simulink model "pillow"  (Simulink 7.0)
settings: Solver=ode45  StartTime=0.0  StopTime=10.0  RelTol=1e-3
settings Model: Creator=FHUANG  LastModifiedBy=FHUANG

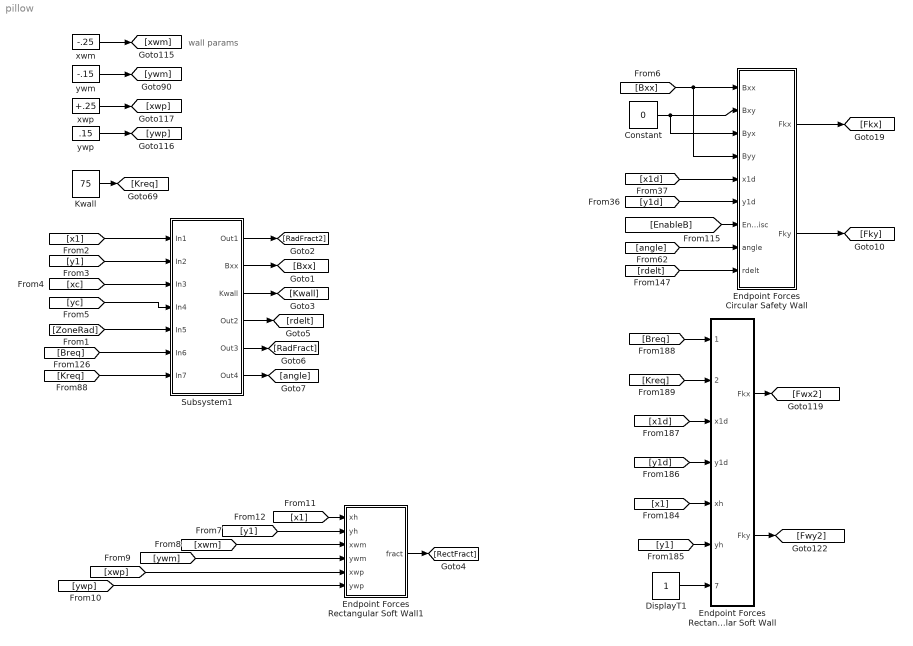
== system pillow ==
  note: wall params
  Constant : Constant  Value=0  OutDataType=sfix(16)  OutScaling=2^0
  DisplayT1 : Constant  OutDataType=sfix(16)  OutScaling=2^0
  Endpoint Forces Circular Safety Wall : Subsystem
  Endpoint Forces Rectangular Soft Wall : Subsystem
  Endpoint Forces Rectangular Soft Wall1 : Subsystem
  Kwall : Constant  Value=75  OutDataType=sfix(16)  OutScaling=2^0
  Subsystem1 : Subsystem
  xwm : Constant  Value=-.25  OutDataType=sfix(16)  OutScaling=2^0
  xwp : Constant  Value=+.25  OutDataType=sfix(16)  OutScaling=2^0
  ywm : Constant  Value=-.15  OutDataType=sfix(16)  OutScaling=2^0
  ywp : Constant  Value=.15  OutDataType=sfix(16)  OutScaling=2^0
  wires:
  [Breq] -> Subsystem1/6(In6)
  [Kreq] -> Subsystem1/7(In7)
  [x1] -> Subsystem1/1(In1)
  [y1] -> Subsystem1/2(In2)
  [xc] -> Subsystem1/3(In3)
  [yc] -> Subsystem1/4(In4)
  [ZoneRad] -> Subsystem1/5(In5)
  Subsystem1/1(Out1) -> [RadFract2]
  Endpoint Forces Circular Safety Wall/1(Fkx) -> [Fkx]
  Endpoint Forces Circular Safety Wall/2(Fky) -> [Fky]
  [Bxx] -> Endpoint Forces Circular Safety Wall/1(Bxx), Endpoint Forces Circular Safety Wall/4(Byy)
  [x1d] -> Endpoint Forces Circular Safety Wall/5(x1d)
  [y1d] -> Endpoint Forces Circular Safety Wall/6(y1d)
  [EnableB] -> Endpoint Forces Circular Safety Wall/7(Enable Visc)
  [angle] -> Endpoint Forces Circular Safety Wall/8(angle)
  [rdelt] -> Endpoint Forces Circular Safety Wall/9(rdelt)
  Constant/1 -> Endpoint Forces Circular Safety Wall/2(Bxy), Endpoint Forces Circular Safety Wall/3(Byx)
  [Breq] -> Endpoint Forces Rectangular Soft Wall/1(Bwall)
  [x1d] -> Endpoint Forces Rectangular Soft Wall/3(x1d)
  [y1d] -> Endpoint Forces Rectangular Soft Wall/4(y1d)
  [x1] -> Endpoint Forces Rectangular Soft Wall/5(xh)
  [Kreq] -> Endpoint Forces Rectangular Soft Wall/2(Kwall)
  Endpoint Forces Rectangular Soft Wall/1(Fkx) -> [Fwx2]
  Endpoint Forces Rectangular Soft Wall/2(Fky) -> [Fwy2]
  ywp/1 -> [ywp]
  xwp/1 -> [xwp]
  xwm/1 -> [xwm]
  ywm/1 -> [ywm]
  Kwall/1 -> [Kreq]
  Subsystem1/2(Bxx) -> [Bxx]
  Subsystem1/3(Kwall) -> [Kwall]
  [x1] -> Endpoint Forces Rectangular Soft Wall1/1(xh)
  [y1] -> Endpoint Forces Rectangular Soft Wall1/2(yh)
  [xwm] -> Endpoint Forces Rectangular Soft Wall1/3(xwm)
  [ywm] -> Endpoint Forces Rectangular Soft Wall1/4(ywm)
  [xwp] -> Endpoint Forces Rectangular Soft Wall1/5(xwp)
  [ywp] -> Endpoint Forces Rectangular Soft Wall1/6(ywp)
  Endpoint Forces Rectangular Soft Wall1/1(fract) -> [RectFract]
  [y1] -> Endpoint Forces Rectangular Soft Wall/6(yh)
  DisplayT1/1 -> Endpoint Forces Rectangular Soft Wall/7(EnableV)
  Subsystem1/4(Out2) -> [rdelt]
  Subsystem1/5(Out3) -> [RadFract]
  Subsystem1/6(Out4) -> [angle]

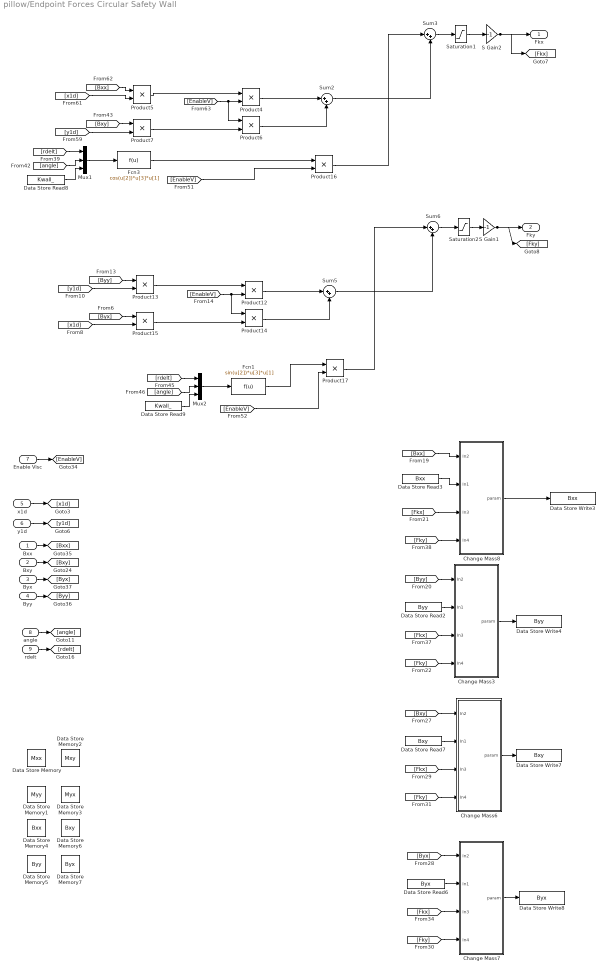
== system pillow/Endpoint Forces Circular Safety Wall ==
  Bxx : Inport  OutDataType=sfix(16)  OutScaling=2^0
  Bxy : Inport  Port=2  OutDataType=sfix(16)  OutScaling=2^0
  Byx : Inport  Port=3  OutDataType=sfix(16)  OutScaling=2^0
  Byy : Inport  Port=4  OutDataType=sfix(16)  OutScaling=2^0
  x1d : Inport  Port=5  OutDataType=sfix(16)  OutScaling=2^0
  y1d : Inport  Port=6  OutDataType=sfix(16)  OutScaling=2^0
  Enable Visc : Inport  Port=7  OutDataType=sfix(16)  OutScaling=2^0
  angle : Inport  Port=8  OutDataType=sfix(16)  OutScaling=2^0
  rdelt : Inport  Port=9  OutDataType=sfix(16)  OutScaling=2^0
  Change Mass3 : Subsystem
  Change Mass6 : Subsystem
  Change Mass7 : Subsystem
  Change Mass8 : Subsystem
  Data Store Memory : DataStoreMemory  DataStoreName=Mxx  OutDataType=sfix(16)  OutScaling=2^0
  Data Store Memory1 : DataStoreMemory  DataStoreName=Myy  OutDataType=sfix(16)  OutScaling=2^0
  Data Store Memory2 : DataStoreMemory  DataStoreName=Mxy  OutDataType=sfix(16)  OutScaling=2^0
  Data Store Memory3 : DataStoreMemory  DataStoreName=Myx  OutDataType=sfix(16)  OutScaling=2^0
  Data Store Memory4 : DataStoreMemory  DataStoreName=Bxx  OutDataType=sfix(16)  OutScaling=2^0
  Data Store Memory5 : DataStoreMemory  DataStoreName=Byy  OutDataType=sfix(16)  OutScaling=2^0
  Data Store Memory6 : DataStoreMemory  DataStoreName=Bxy  OutDataType=sfix(16)  OutScaling=2^0
  Data Store Memory7 : DataStoreMemory  DataStoreName=Byx  OutDataType=sfix(16)  OutScaling=2^0
  Data Store Read2 : DataStoreRead  DataStoreName=Byy  SampleTime=0
  Data Store Read3 : DataStoreRead  DataStoreName=Bxx  SampleTime=0
  Data Store Read6 : DataStoreRead  DataStoreName=Byx  SampleTime=0
  Data Store Read7 : DataStoreRead  DataStoreName=Bxy  SampleTime=0
  Data Store Read8 : DataStoreRead  DataStoreName=Kwall_  SampleTime=0
  Data Store Read9 : DataStoreRead  DataStoreName=Kwall_  SampleTime=0
  Data Store Write3 : DataStoreWrite  DataStoreName=Bxx  SampleTime=-1
  Data Store Write4 : DataStoreWrite  DataStoreName=Byy  SampleTime=-1
  Data Store Write7 : DataStoreWrite  DataStoreName=Bxy  SampleTime=-1
  Data Store Write8 : DataStoreWrite  DataStoreName=Byx  SampleTime=-1
  Fcn1 : Fcn  Expr=sin(u[2])*u[3]*u[1]
  Fcn3 : Fcn  Expr=cos(u[2])*u[3]*u[1]
  Mux1 : Mux  Inputs=3
  Mux2 : Mux  Inputs=3
  Product{4..7,12..17} (10 alike) : Product  OutDataType=sfix(16)  OutScaling=2^0  RndMeth=Zero
  S Gain1 : Gain  Gain=-1  ParameterDataType=sfix(16)  ParameterScaling=2^0  OutDataType=sfix(16)  OutScaling=2^0  SaturateOnIntegerOverflow=on
  S Gain2 : Gain  Gain=-1  ParameterDataType=sfix(16)  ParameterScaling=2^0  OutDataType=sfix(16)  OutScaling=2^0  SaturateOnIntegerOverflow=on
  Saturation1 : Saturate  UpperLimit=80  LowerLimit=-80
  Saturation2 : Saturate  UpperLimit=80  LowerLimit=-80
  Sum{2..3,5..6} (4 alike) : Sum  Inputs=|++  OutDataType=sfix(16)  OutScaling=2^0
  Fkx : Outport  OutDataType=sfix(16)  OutScaling=2^0
  Fky : Outport  Port=2  OutDataType=sfix(16)  OutScaling=2^0
  wires:
  Product5/1 -> Product4/1
  [EnableV] -> Product6/1, Product4/2
  Product4/1 -> Sum2/1
  Product6/1 -> Sum2/2
  Product7/1 -> Product6/2
  Sum3/1 -> Saturation1/1
  [Bxx] -> Product5/1
  [x1d] -> Product5/2
  Bxx/1 -> [Bxx]
  [Bxy] -> Product7/1
  [y1d] -> Product7/2
  Bxy/1 -> [Bxy]
  Byx/1 -> [Byx]
  Byy/1 -> [Byy]
  x1d/1 -> [x1d]
  y1d/1 -> [y1d]
  Enable Visc/1 -> [EnableV]
  Product13/1 -> Product12/1
  [EnableV] -> Product12/2, Product14/1
  Product12/1 -> Sum5/1
  Product14/1 -> Sum5/2
  Product15/1 -> Product14/2
  [Byy] -> Product13/1
  [y1d] -> Product13/2
  [Byx] -> Product15/1
  [x1d] -> Product15/2
  S Gain2/1 -> Fkx/1, [Fkx]
  Saturation1/1 -> S Gain2/1
  Saturation2/1 -> S Gain1/1
  Sum6/1 -> Saturation2/1
  S Gain1/1 -> Fky/1, [Fky]
  Change Mass8/1(param) -> Data Store Write3/1
  Change Mass3/1(param) -> Data Store Write4/1
  [Byy] -> Change Mass3/1(In2)
  Data Store Read2/1 -> Change Mass3/2(In1)
  [Fky] -> Change Mass3/4(In4)
  Change Mass6/1(param) -> Data Store Write7/1
  [Bxy] -> Change Mass6/1(In2)
  Data Store Read7/1 -> Change Mass6/2(In1)
  [Fkx] -> Change Mass6/3(In3)
  Change Mass7/1(param) -> Data Store Write8/1
  [Byx] -> Change Mass7/1(In2)
  Data Store Read6/1 -> Change Mass7/2(In1)
  [Fky] -> Change Mass7/4(In4)
  [Fky] -> Change Mass6/4(In4)
  [Fkx] -> Change Mass7/3(In3)
  [Fkx] -> Change Mass3/3(In3)
  [Bxx] -> Change Mass8/1(In2)
  Data Store Read3/1 -> Change Mass8/2(In1)
  [Fkx] -> Change Mass8/3(In3)
  [Fky] -> Change Mass8/4(In4)
  Sum2/1 -> Sum3/2
  Sum5/1 -> Sum6/2
  [rdelt] -> Mux1/1
  [angle] -> Mux1/2
  Mux1/1 -> Fcn3/1
  [rdelt] -> Mux2/1
  [angle] -> Mux2/2
  Mux2/1 -> Fcn1/1
  Data Store Read8/1 -> Mux1/3
  Product16/1 -> Sum3/1
  Product17/1 -> Sum6/1
  Data Store Read9/1 -> Mux2/3
  Fcn1/1 -> Product17/1
  Fcn3/1 -> Product16/1
  [EnableV] -> Product16/2
  [EnableV] -> Product17/2
  angle/1 -> [angle]
  rdelt/1 -> [rdelt]

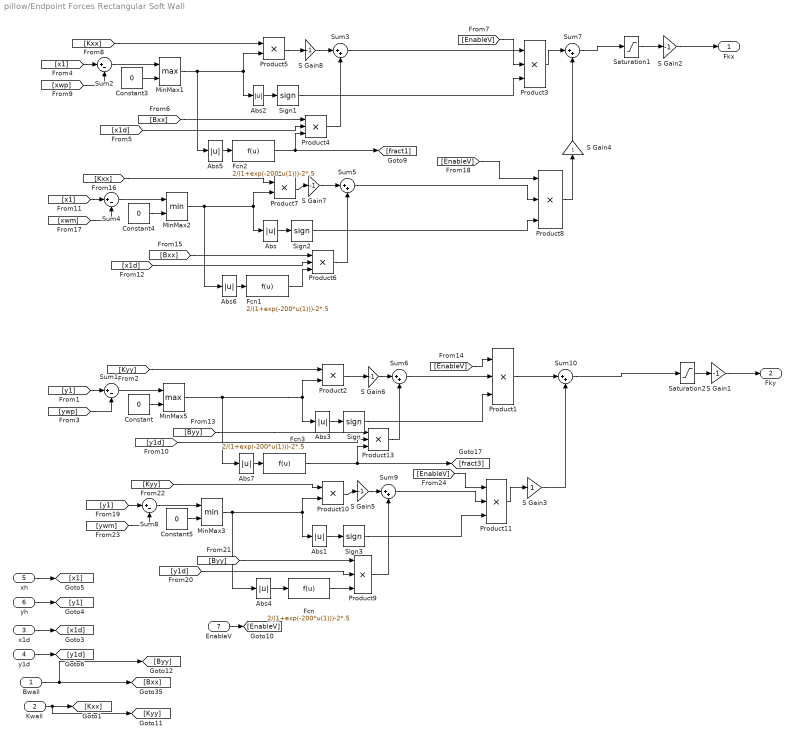
== system pillow/Endpoint Forces Rectangular Soft Wall ==
  Bwall : Inport  OutDataType=sfix(16)  OutScaling=2^0
  Kwall : Inport  Port=2  OutDataType=sfix(16)  OutScaling=2^0
  x1d : Inport  Port=3  OutDataType=sfix(16)  OutScaling=2^0
  y1d : Inport  Port=4  OutDataType=sfix(16)  OutScaling=2^0
  xh : Inport  Port=5  OutDataType=sfix(16)  OutScaling=2^0
  yh : Inport  Port=6  OutDataType=sfix(16)  OutScaling=2^0
  EnableV : Inport  Port=7  OutDataType=sfix(16)  OutScaling=2^0
  Abs{,1..7} (8 alike) : Abs
  Constant{,3..5} (4 alike) : Constant  Value=0  OutDataType=sfix(16)  OutScaling=2^0
  Fcn{,1..3} (4 alike) : Fcn  Expr=2/(1+exp(-200*u(1)))-2*.5
  MinMax1 : MinMax  Function=max  Inputs=2  OutDataType=sfix(16)  OutScaling=2^0
  MinMax2 : MinMax  Inputs=2  OutDataType=sfix(16)  OutScaling=2^0
  MinMax3 : MinMax  Inputs=2  OutDataType=sfix(16)  OutScaling=2^0
  MinMax5 : MinMax  Function=max  Inputs=2  OutDataType=sfix(16)  OutScaling=2^0
  Product{1,3..4,6,8..9,11,13} (8 alike) : Product  Inputs=3  OutDataType=sfix(16)  OutScaling=2^0  RndMeth=Zero
  Product{2,5,7,10} (4 alike) : Product  OutDataType=sfix(16)  OutScaling=2^0  RndMeth=Zero
  S Gain{1..2,5..8} (6 alike) : Gain  Gain=-1  ParameterDataType=sfix(16)  ParameterScaling=2^0  OutDataType=sfix(16)  OutScaling=2^0  SaturateOnIntegerOverflow=on
  S Gain3 : Gain  ParameterDataType=sfix(16)  ParameterScaling=2^0  OutDataType=sfix(16)  OutScaling=2^0  SaturateOnIntegerOverflow=on
  S Gain4 : Gain  Orientation=up  ParameterDataType=sfix(16)  ParameterScaling=2^0  OutDataType=sfix(16)  OutScaling=2^0  SaturateOnIntegerOverflow=on
  Saturation1 : Saturate  UpperLimit=80  LowerLimit=-80
  Saturation2 : Saturate  UpperLimit=80  LowerLimit=-80
  Sign{,1..3} (4 alike) : Signum
  Sum{1..2,4,8} (4 alike) : Sum  Inputs=|+-  OutDataType=sfix(16)  OutScaling=2^0
  Sum{3,5..7,9..10} (6 alike) : Sum  Inputs=|++  OutDataType=sfix(16)  OutScaling=2^0
  Fkx : Outport  OutDataType=sfix(16)  OutScaling=2^0
  Fky : Outport  Port=2  OutDataType=sfix(16)  OutScaling=2^0
  wires:
  S Gain1/1 -> Fky/1
  Saturation2/1 -> S Gain1/1
  Saturation1/1 -> S Gain2/1
  S Gain2/1 -> Fkx/1
  y1d/1 -> [y1d]
  x1d/1 -> [x1d]
  Bwall/1 -> [Bxx], [Byy]
  Kwall/1 -> [Kxx], [Kyy]
  yh/1 -> [y1]
  xh/1 -> [x1]
  [y1d] -> Product13/2
  [Byy] -> Product13/1
  Product13/1 -> Sum6/2
  [EnableV] -> Product1/1
  Sum6/1 -> Product1/2
  [Kyy] -> Product2/1
  Product2/1 -> S Gain6/1
  Sign/1 -> Product1/3
  [x1d] -> Product4/2
  [Bxx] -> Product4/1
  Product4/1 -> Sum3/2
  [EnableV] -> Product3/1
  Sum3/1 -> Product3/2
  [Kxx] -> Product5/1
  [x1] -> Sum2/1
  Sum2/1 -> MinMax1/1
  [xwp] -> Sum2/2
  Product5/1 -> S Gain8/1
  Constant3/1 -> MinMax1/2
  MinMax1/1 -> Product5/2, Abs2/1, Abs5/1
  Sign1/1 -> Product3/3
  EnableV/1 -> [EnableV]
  [x1d] -> Product6/2
  [Bxx] -> Product6/1
  Product6/1 -> Sum5/2
  Sum5/1 -> Product8/2
  [Kxx] -> Product7/1
  [x1] -> Sum4/1
  Sum4/1 -> MinMax2/1
  [xwm] -> Sum4/2
  Product7/1 -> S Gain7/1
  Constant4/1 -> MinMax2/2
  MinMax2/1 -> Product7/2, Abs/1, Abs6/1
  Sign2/1 -> Product8/3
  [EnableV] -> Product8/1
  Product3/1 -> Sum7/1
  Sum7/1 -> Saturation1/1
  Product8/1 -> S Gain4/1
  Abs/1 -> Sign2/1
  [y1d] -> Product9/2
  [Byy] -> Product9/1
  Product9/1 -> Sum9/2
  Sum9/1 -> Product11/2
  [Kyy] -> Product10/1
  [y1] -> Sum8/1
  Sum8/1 -> MinMax3/1
  [ywm] -> Sum8/2
  Product10/1 -> S Gain5/1
  Constant5/1 -> MinMax3/2
  MinMax3/1 -> Product10/2, Abs1/1, Abs4/1
  Sign3/1 -> Product11/3
  [EnableV] -> Product11/1
  Product1/1 -> Sum10/1
  Product11/1 -> S Gain3/1
  Sum10/1 -> Saturation2/1
  Abs1/1 -> Sign3/1
  Abs2/1 -> Sign1/1
  Abs3/1 -> Sign/1
  S Gain3/1 -> Sum10/2
  S Gain4/1 -> Sum7/2
  S Gain5/1 -> Sum9/1
  S Gain6/1 -> Sum6/1
  S Gain7/1 -> Sum5/1
  S Gain8/1 -> Sum3/1
  Abs4/1 -> Fcn/1
  Abs6/1 -> Fcn1/1
  Abs5/1 -> Fcn2/1
  Fcn2/1 -> Product4/3, [fract1]
  Fcn/1 -> Product9/3
  Fcn1/1 -> Product6/3
  Abs7/1 -> Fcn3/1
  Fcn3/1 -> Product13/3, [fract3]
  [y1] -> Sum1/1
  Sum1/1 -> MinMax5/1
  [ywp] -> Sum1/2
  Constant/1 -> MinMax5/2
  MinMax5/1 -> Product2/2, Abs3/1, Abs7/1

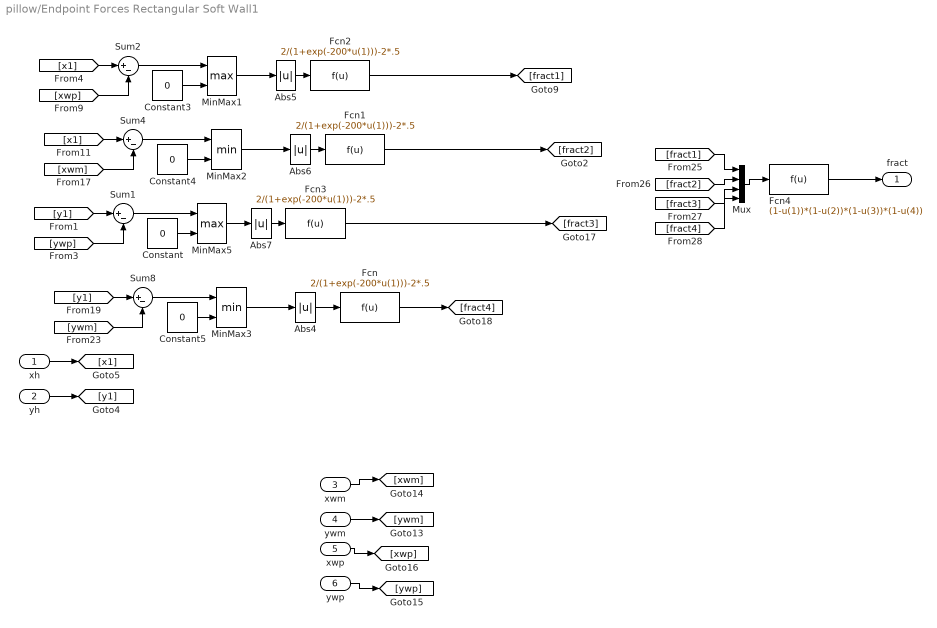
== system pillow/Endpoint Forces Rectangular Soft Wall1 ==
  xh : Inport  OutDataType=sfix(16)  OutScaling=2^0
  yh : Inport  Port=2  OutDataType=sfix(16)  OutScaling=2^0
  xwm : Inport  Port=3  OutDataType=sfix(16)  OutScaling=2^0
  ywm : Inport  Port=4  OutDataType=sfix(16)  OutScaling=2^0
  xwp : Inport  Port=5  OutDataType=sfix(16)  OutScaling=2^0
  ywp : Inport  Port=6  OutDataType=sfix(16)  OutScaling=2^0
  Abs{4..7} (4 alike) : Abs
  Constant{,3..5} (4 alike) : Constant  Value=0  OutDataType=sfix(16)  OutScaling=2^0
  Fcn{,1..3} (4 alike) : Fcn  Expr=2/(1+exp(-200*u(1)))-2*.5
  Fcn4 : Fcn  Expr=(1-u(1))*(1-u(2))*(1-u(3))*(1-u(4))
  MinMax1 : MinMax  Function=max  Inputs=2  OutDataType=sfix(16)  OutScaling=2^0
  MinMax2 : MinMax  Inputs=2  OutDataType=sfix(16)  OutScaling=2^0
  MinMax3 : MinMax  Inputs=2  OutDataType=sfix(16)  OutScaling=2^0
  MinMax5 : MinMax  Function=max  Inputs=2  OutDataType=sfix(16)  OutScaling=2^0
  Mux : Mux
  Sum{1..2,4,8} (4 alike) : Sum  Inputs=|+-  OutDataType=sfix(16)  OutScaling=2^0
  fract : Outport  OutDataType=sfix(16)  OutScaling=2^0
  wires:
  yh/1 -> [y1]
  xh/1 -> [x1]
  [y1] -> Sum1/1
  Sum1/1 -> MinMax5/1
  [ywp] -> Sum1/2
  Constant/1 -> MinMax5/2
  MinMax5/1 -> Abs7/1
  [x1] -> Sum2/1
  Sum2/1 -> MinMax1/1
  [xwp] -> Sum2/2
  Constant3/1 -> MinMax1/2
  MinMax1/1 -> Abs5/1
  [x1] -> Sum4/1
  Sum4/1 -> MinMax2/1
  [xwm] -> Sum4/2
  Constant4/1 -> MinMax2/2
  MinMax2/1 -> Abs6/1
  [y1] -> Sum8/1
  Sum8/1 -> MinMax3/1
  [ywm] -> Sum8/2
  Constant5/1 -> MinMax3/2
  MinMax3/1 -> Abs4/1
  Abs4/1 -> Fcn/1
  Abs6/1 -> Fcn1/1
  Abs5/1 -> Fcn2/1
  Fcn2/1 -> [fract1]
  Fcn/1 -> [fract4]
  Fcn1/1 -> [fract2]
  Abs7/1 -> Fcn3/1
  Fcn3/1 -> [fract3]
  xwm/1 -> [xwm]
  ywm/1 -> [ywm]
  xwp/1 -> [xwp]
  ywp/1 -> [ywp]
  [fract1] -> Mux/1
  [fract2] -> Mux/2
  [fract3] -> Mux/3
  [fract4] -> Mux/4
  Mux/1 -> Fcn4/1
  Fcn4/1 -> fract/1

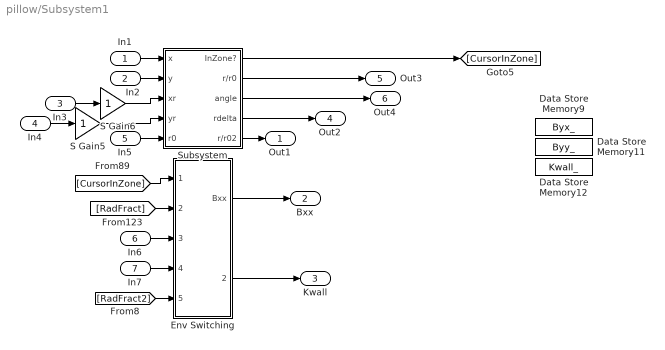
== system pillow/Subsystem1 ==
  In1 : Inport
  In2 : Inport  Port=2
  In3 : Inport  Port=3
  In4 : Inport  Port=4
  In5 : Inport  Port=5
  In6 : Inport  Port=6
  In7 : Inport  Port=7
  Data Store Memory11 : DataStoreMemory  DataStoreName=Byy_  OutDataType=sfix(16)  OutScaling=2^0
  Data Store Memory12 : DataStoreMemory  DataStoreName=Kwall_  OutDataType=sfix(16)  OutScaling=2^0
  Data Store Memory9 : DataStoreMemory  DataStoreName=Byx_  OutDataType=sfix(16)  OutScaling=2^0
  "Env Switching " : Subsystem
  S Gain5 : Gain  ParameterDataType=sfix(16)  ParameterScaling=2^0  OutDataType=sfix(16)  OutScaling=2^0  SaturateOnIntegerOverflow=on
  S Gain6 : Gain  ParameterDataType=sfix(16)  ParameterScaling=2^0  OutDataType=sfix(16)  OutScaling=2^0  SaturateOnIntegerOverflow=on
  Subsystem : Subsystem
  Out1 : Outport
  Bxx : Outport  Port=2  OutDataType=sfix(16)  OutScaling=2^0
  Kwall : Outport  Port=3  OutDataType=sfix(16)  OutScaling=2^0
  Out2 : Outport  Port=4
  Out3 : Outport  Port=5
  Out4 : Outport  Port=6
  wires:
  [CursorInZone] -> "Env Switching "/1(Inzone)
  [RadFract] -> "Env Switching "/2(RadFact)
  [RadFract2] -> "Env Switching "/5(RadFract2)
  Subsystem/1(InZone?) -> [CursorInZone]
  S Gain5/1 -> Subsystem/4(yr)
  S Gain6/1 -> Subsystem/3(xr)
  Subsystem/4(rdelta) -> Out2/1
  Subsystem/3(angle) -> Out4/1
  In1/1 -> Subsystem/1(x)
  In2/1 -> Subsystem/2(y)
  In3/1 -> S Gain6/1
  In4/1 -> S Gain5/1
  In5/1 -> Subsystem/5(r0)
  Subsystem/5(r/r02) -> Out1/1
  In6/1 -> "Env Switching "/3(B_out)
  In7/1 -> "Env Switching "/4(K_out)
  "Env Switching "/1(Bxx) -> Bxx/1
  "Env Switching "/2(Kwall) -> Kwall/1
  Subsystem/2(r/r0) -> Out3/1

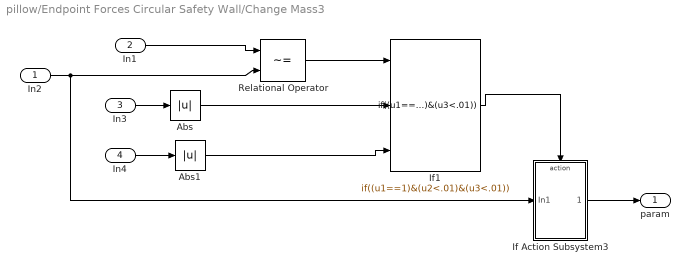
== system pillow/Endpoint Forces Circular Safety Wall/Change Mass3 ==
  In2 : Inport  OutDataType=sfix(16)  OutScaling=2^0
  In1 : Inport  Port=2  OutDataType=sfix(16)  OutScaling=2^0
  In3 : Inport  Port=3  OutDataType=sfix(16)  OutScaling=2^0
  In4 : Inport  Port=4  OutDataType=sfix(16)  OutScaling=2^0
  Abs : Abs
  Abs1 : Abs
  If Action Subsystem3 : Subsystem  TreatAsAtomicUnit=on
  If1 : If  NumInputs=3  IfExpression=(u1==1)&(u2<.01)&(u3<.01)  ShowElse=off
  Relational Operator : RelationalOperator  Operator=~=  InputSameDT=on
  param : Outport  OutDataType=sfix(16)  OutScaling=2^0
  wires:
  Relational Operator/1 -> If1/1
  If1/1 -> If Action Subsystem3/Action
  In2/1 -> If Action Subsystem3/1(In1), Relational Operator/2
  In1/1 -> Relational Operator/1
  If Action Subsystem3/1(Output Angle) -> param/1
  In4/1 -> Abs1/1
  In3/1 -> Abs/1
  Abs/1 -> If1/2
  Abs1/1 -> If1/3

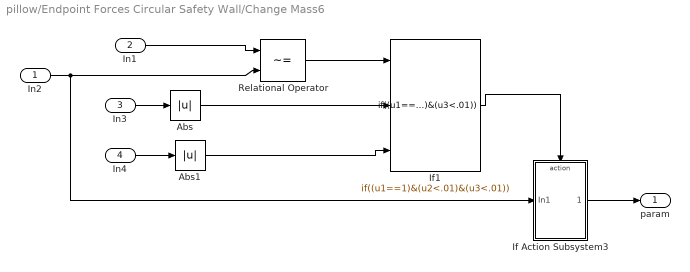
== system pillow/Endpoint Forces Circular Safety Wall/Change Mass6 ==
  In2 : Inport  OutDataType=sfix(16)  OutScaling=2^0
  In1 : Inport  Port=2  OutDataType=sfix(16)  OutScaling=2^0
  In3 : Inport  Port=3  OutDataType=sfix(16)  OutScaling=2^0
  In4 : Inport  Port=4  OutDataType=sfix(16)  OutScaling=2^0
  Abs : Abs
  Abs1 : Abs
  If Action Subsystem3 : Subsystem  TreatAsAtomicUnit=on
  If1 : If  NumInputs=3  IfExpression=(u1==1)&(u2<.01)&(u3<.01)  ShowElse=off
  Relational Operator : RelationalOperator  Operator=~=  InputSameDT=on
  param : Outport  OutDataType=sfix(16)  OutScaling=2^0
  wires:
  Relational Operator/1 -> If1/1
  If1/1 -> If Action Subsystem3/Action
  In2/1 -> If Action Subsystem3/1(In1), Relational Operator/2
  In1/1 -> Relational Operator/1
  If Action Subsystem3/1(Output Angle) -> param/1
  In4/1 -> Abs1/1
  In3/1 -> Abs/1
  Abs/1 -> If1/2
  Abs1/1 -> If1/3

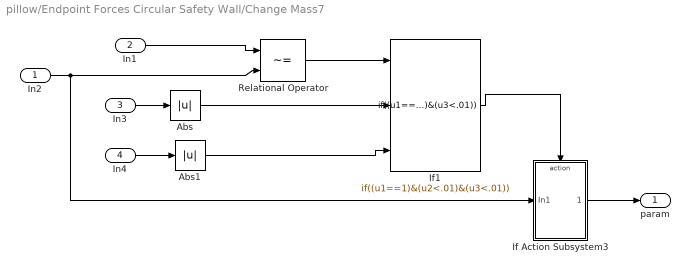
== system pillow/Endpoint Forces Circular Safety Wall/Change Mass7 ==
  In2 : Inport  OutDataType=sfix(16)  OutScaling=2^0
  In1 : Inport  Port=2  OutDataType=sfix(16)  OutScaling=2^0
  In3 : Inport  Port=3  OutDataType=sfix(16)  OutScaling=2^0
  In4 : Inport  Port=4  OutDataType=sfix(16)  OutScaling=2^0
  Abs : Abs
  Abs1 : Abs
  If Action Subsystem3 : Subsystem  TreatAsAtomicUnit=on
  If1 : If  NumInputs=3  IfExpression=(u1==1)&(u2<.01)&(u3<.01)  ShowElse=off
  Relational Operator : RelationalOperator  Operator=~=  InputSameDT=on
  param : Outport  OutDataType=sfix(16)  OutScaling=2^0
  wires:
  Abs1/1 -> If1/3
  Abs/1 -> If1/2
  In3/1 -> Abs/1
  In4/1 -> Abs1/1
  If Action Subsystem3/1(Output Angle) -> param/1
  In1/1 -> Relational Operator/1
  In2/1 -> Relational Operator/2, If Action Subsystem3/1(In1)
  If1/1 -> If Action Subsystem3/Action
  Relational Operator/1 -> If1/1

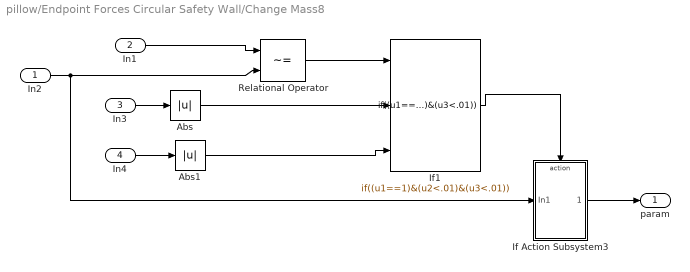
== system pillow/Endpoint Forces Circular Safety Wall/Change Mass8 ==
  In2 : Inport  OutDataType=sfix(16)  OutScaling=2^0
  In1 : Inport  Port=2  OutDataType=sfix(16)  OutScaling=2^0
  In3 : Inport  Port=3  OutDataType=sfix(16)  OutScaling=2^0
  In4 : Inport  Port=4  OutDataType=sfix(16)  OutScaling=2^0
  Abs : Abs
  Abs1 : Abs
  If Action Subsystem3 : Subsystem  TreatAsAtomicUnit=on
  If1 : If  NumInputs=3  IfExpression=(u1==1)&(u2<.01)&(u3<.01)  ShowElse=off
  Relational Operator : RelationalOperator  Operator=~=  InputSameDT=on
  param : Outport  OutDataType=sfix(16)  OutScaling=2^0
  wires:
  Abs1/1 -> If1/3
  Abs/1 -> If1/2
  In3/1 -> Abs/1
  In4/1 -> Abs1/1
  If Action Subsystem3/1(Output Angle) -> param/1
  In1/1 -> Relational Operator/1
  In2/1 -> Relational Operator/2, If Action Subsystem3/1(In1)
  If1/1 -> If Action Subsystem3/Action
  Relational Operator/1 -> If1/1

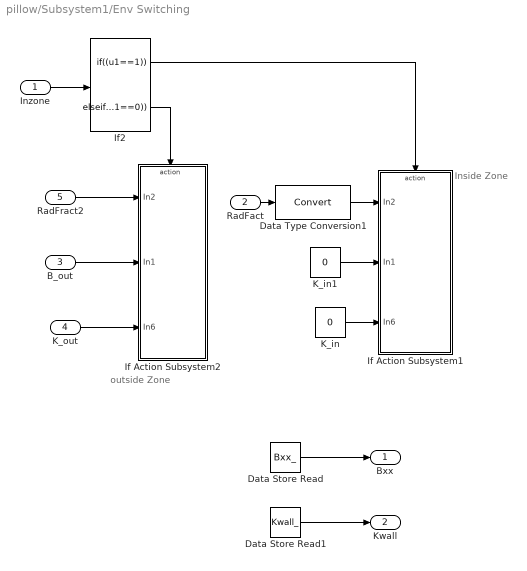
== system pillow/Subsystem1/Env Switching  ==
  note: outside Zone
  note: Inside Zone
  Inzone : Inport  OutDataType=sfix(16)  OutScaling=2^0
  RadFact : Inport  Port=2  OutDataType=sfix(16)  OutScaling=2^0
  B_out : Inport  Port=3  OutDataType=sfix(16)  OutScaling=2^0
  K_out : Inport  Port=4  OutDataType=sfix(16)  OutScaling=2^0
  RadFract2 : Inport  Port=5  OutDataType=sfix(16)  OutScaling=2^0
  Data Store Read : DataStoreRead  DataStoreName=Bxx_  SampleTime=0
  Data Store Read1 : DataStoreRead  DataStoreName=Kwall_  SampleTime=0
  Data Type Conversion1 : DataTypeConversion  OutDataType=sfix(16)  OutScaling=2^0
  If Action Subsystem1 : Subsystem  TreatAsAtomicUnit=on
  If Action Subsystem2 : Subsystem  TreatAsAtomicUnit=on
  If2 : If  IfExpression=(u1==1)  ElseIfExpressions=(u1==0)  ShowElse=off
  K_in : Constant  Value=0  OutDataType=sfix(16)  OutScaling=2^0
  K_in1 : Constant  Value=0  OutDataType=sfix(16)  OutScaling=2^0
  Bxx : Outport  OutDataType=sfix(16)  OutScaling=2^0
  Kwall : Outport  Port=2  OutDataType=sfix(16)  OutScaling=2^0
  wires:
  If2/1 -> If Action Subsystem1/Action
  Inzone/1 -> If2/1
  If2/2 -> If Action Subsystem2/Action
  RadFact/1 -> Data Type Conversion1/1
  Data Type Conversion1/1 -> If Action Subsystem1/1(In2)
  B_out/1 -> If Action Subsystem2/2(In1)
  K_out/1 -> If Action Subsystem2/3(In6)
  K_in/1 -> If Action Subsystem1/3(In6)
  RadFract2/1 -> If Action Subsystem2/1(In2)
  K_in1/1 -> If Action Subsystem1/2(In1)
  Data Store Read/1 -> Bxx/1
  Data Store Read1/1 -> Kwall/1

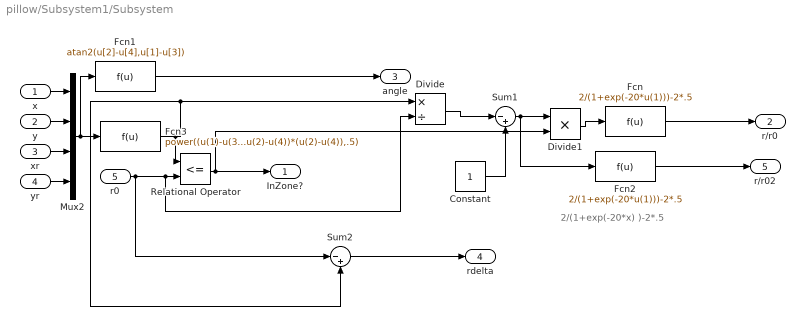
== system pillow/Subsystem1/Subsystem ==
  note: 2/(1+exp(-20*x) )-2*.5
  x : Inport  OutDataType=sfix(16)  OutScaling=2^0
  y : Inport  Port=2  OutDataType=sfix(16)  OutScaling=2^0
  xr : Inport  Port=3  OutDataType=sfix(16)  OutScaling=2^0
  yr : Inport  Port=4  OutDataType=sfix(16)  OutScaling=2^0
  r0 : Inport  Port=5  OutDataType=sfix(16)  OutScaling=2^0
  Constant : Constant  OutDataType=sfix(16)  OutScaling=2^0
  Divide : Product  Inputs=*/  OutDataType=sfix(16)  OutScaling=2^-10
  Divide1 : Product  Inputs=**  OutDataType=sfix(16)  OutScaling=2^-10
  Fcn : Fcn  Expr=2/(1+exp(-20*u(1)))-2*.5
  Fcn1 : Fcn  Expr=atan2(u[2]-u[4],u[1]-u[3])
  Fcn2 : Fcn  Expr=2/(1+exp(-20*u(1)))-2*.5
  Fcn3 : Fcn  Expr=power((u(1)-u(3))*(u(1)-u(3))+(u(2)-u(4))*(u(2)-u(4)),.5)
  Mux2 : Mux
  Relational Operator : RelationalOperator  Operator=<=  LogicOutDataTypeMode=boolean
  Sum1 : Sum  Inputs=|-+  OutDataType=sfix(16)  OutScaling=2^0
  Sum2 : Sum  Inputs=|-+  OutDataType=sfix(16)  OutScaling=2^0
  InZone? : Outport  OutDataType=sfix(16)  OutScaling=2^0
  r/r0 : Outport  Port=2  OutDataType=sfix(16)  OutScaling=2^0
  angle : Outport  Port=3  OutDataType=sfix(16)  OutScaling=2^0
  rdelta : Outport  Port=4  OutDataType=sfix(16)  OutScaling=2^0
  r/r02 : Outport  Port=5  OutDataType=sfix(16)  OutScaling=2^0
  wires:
  Mux2/1 -> Fcn3/1, Fcn1/1
  Fcn3/1 -> Relational Operator/1, Divide/1, Sum2/2
  x/1 -> Mux2/1
  y/1 -> Mux2/2
  xr/1 -> Mux2/3
  Relational Operator/1 -> InZone?/1, Divide1/2
  r0/1 -> Relational Operator/2, Divide/2, Sum2/1
  yr/1 -> Mux2/4
  Divide/1 -> Sum1/1
  Constant/1 -> Sum1/2
  Sum1/1 -> Divide1/1, Fcn2/1
  Divide1/1 -> Fcn/1
  Fcn/1 -> r/r0/1
  Fcn1/1 -> angle/1
  Sum2/1 -> rdelta/1
  Fcn2/1 -> r/r02/1

== system pillow/Endpoint Forces Circular Safety Wall/Change Mass3/If Action Subsystem3 ==
  In1 : Inport  OutDataType=sfix(16)  OutScaling=2^0
  Action Port : ActionPort
  Output Angle : Outport  OutDataType=sfix(16)  OutScaling=2^0
  wires:
  In1/1 -> Output Angle/1

== system pillow/Endpoint Forces Circular Safety Wall/Change Mass6/If Action Subsystem3 ==
  In1 : Inport  OutDataType=sfix(16)  OutScaling=2^0
  Action Port : ActionPort
  Output Angle : Outport  OutDataType=sfix(16)  OutScaling=2^0
  wires:
  In1/1 -> Output Angle/1

== system pillow/Endpoint Forces Circular Safety Wall/Change Mass7/If Action Subsystem3 ==
  In1 : Inport  OutDataType=sfix(16)  OutScaling=2^0
  Action Port : ActionPort
  Output Angle : Outport  OutDataType=sfix(16)  OutScaling=2^0
  wires:
  In1/1 -> Output Angle/1

== system pillow/Endpoint Forces Circular Safety Wall/Change Mass8/If Action Subsystem3 ==
  In1 : Inport  OutDataType=sfix(16)  OutScaling=2^0
  Action Port : ActionPort
  Output Angle : Outport  OutDataType=sfix(16)  OutScaling=2^0
  wires:
  In1/1 -> Output Angle/1

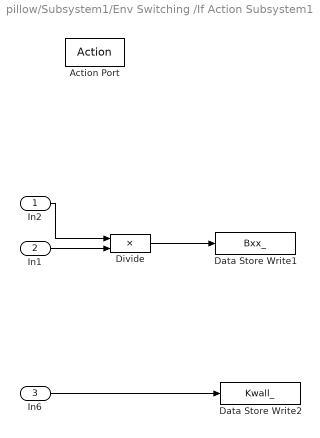
== system pillow/Subsystem1/Env Switching /If Action Subsystem1 ==
  In2 : Inport  OutDataType=sfix(16)  OutScaling=2^0
  In1 : Inport  Port=2  OutDataType=sfix(16)  OutScaling=2^0
  In6 : Inport  Port=3  OutDataType=sfix(16)  OutScaling=2^0
  Action Port : ActionPort
  Data Store Write1 : DataStoreWrite  DataStoreName=Bxx_  SampleTime=-1
  Data Store Write2 : DataStoreWrite  DataStoreName=Kwall_  SampleTime=-1
  Divide : Product  Inputs=**  OutDataType=sfix(16)  OutScaling=2^-10
  wires:
  In2/1 -> Divide/1
  In1/1 -> Divide/2
  Divide/1 -> Data Store Write1/1
  In6/1 -> Data Store Write2/1

== system pillow/Subsystem1/Env Switching /If Action Subsystem2 ==
  In2 : Inport  OutDataType=sfix(16)  OutScaling=2^0
  In1 : Inport  Port=2  OutDataType=sfix(16)  OutScaling=2^0
  In6 : Inport  Port=3  OutDataType=sfix(16)  OutScaling=2^0
  Action Port : ActionPort
  Data Store Write1 : DataStoreWrite  DataStoreName=Bxx_  SampleTime=-1
  Data Store Write2 : DataStoreWrite  DataStoreName=Kwall_  SampleTime=-1
  Divide : Product  Inputs=**  OutDataType=sfix(16)  OutScaling=2^-10
  wires:
  Divide/1 -> Data Store Write1/1
  In1/1 -> Divide/2
  In2/1 -> Divide/1
  In6/1 -> Data Store Write2/1
